simulink model "NLSFS_MODEL"  (Simulink 7.6)
settings: Solver=ode45  StartTime=0.0  StopTime=10  RelTol=1e-3
settings Model: Creator=Administrator  LastModifiedBy=Administrator
settings DebuggingCC: SolverPrmCheckMsg=none

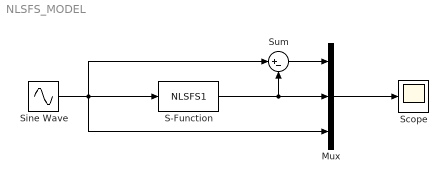
== system NLSFS_MODEL ==
  Mux : Mux  Inputs=3
  S-Function : S-Function  FunctionName=NLSFS1  EnableBusSupport=off
  Scope : Scope
      settings: YMin=-1.1  YMax=0.3
  Sine Wave : Sin  SampleTime=0.01
  Sum : Sum  Inputs=|+-
  wires:
  Sine Wave/1 -> S-Function/1, Sum/1, Mux/3
  S-Function/1 -> Sum/2, Mux/2
  Mux/1 -> Scope/1
  Sum/1 -> Mux/1
